simulink model "examples_of_saturation_block_as_mask"  (R2021a)
settings: Solver=VariableStepAuto  StartTime=0.0  StopTime=10.0  RelTol=1e-3
settings Model: Creator=YasserNet  LastModifiedBy=YasserNet

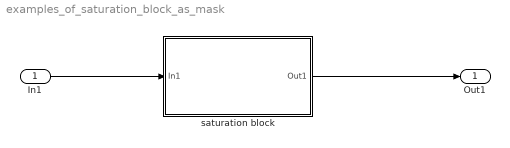
== system examples_of_saturation_block_as_mask ==
  In1 : Inport  mask{u=0, l=0}
      mask prompts: u "upper value"; l "lower value"
      mask DialogControl DescGroupVar Prompt: saturation block
      mask DialogControl DescTextVar Prompt: limit input signal to the upper and lower saturation values
  saturation block : Subsystem  mask{u=0, l=0}
      mask prompts: u "upper"; l "lower"
      mask DialogControl DescGroupVar Prompt: saturation block
      mask DialogControl DescTextVar Prompt: limit input signal to the upper and the lower saturation values
  Out1 : Outport
  wires:
  In1/1 -> saturation block/1(In1)
  saturation block/1(Out1) -> Out1/1

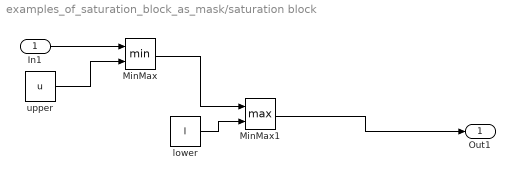
== system examples_of_saturation_block_as_mask/saturation block ==
  In1 : Inport
  MinMax : MinMax  Inputs=2
  MinMax1 : MinMax  Function=max  Inputs=2
  lower : Constant  Value=l
  upper : Constant  Value=u
  Out1 : Outport
  wires:
  MinMax1/1 -> Out1/1
  upper/1 -> MinMax/2
  In1/1 -> MinMax/1
  MinMax/1 -> MinMax1/1
  lower/1 -> MinMax1/2
